simulink library "csu_tfl_thruster_forces_lander_lib"  (R2015b)
settings: Solver=ode45  StartTime=0.0  StopTime=10.0  RelTol=1e-3
values from neighbouring files (symbols this model uses):
  Bm = gim_motor_Bm    [csu_gmb_motor_prep.m]
  Jm = gim_motor_Jm    [csu_gmb_motor_prep.m]
  Ke = gim_motor_Ke    [csu_gmb_motor_prep.m]
  Kl = gim_motor_Kl    [csu_gmb_motor_prep.m]
  Kt = gim_motor_Kt    [csu_gmb_motor_prep.m]
  Lm = gim_motor_Lm    [csu_gmb_motor_prep.m]
  nb = gim_motor_nb    [csu_gmb_motor_prep.m]
  Rm = gim_motor_Rm    [csu_gmb_motor_prep.m]
undefined symbols (not defined in the file or in its folder): DiscIntNeverNeededParam, tpl_x_gimbal_actuator_to_angle, tpl_y_gimbal_actuator_to_angle
libraries: util_thruster_lib x26, util_quat_lib x2, util_info_lib x1
settings Model: Creator=Nilesh  LastModifiedBy=jimkaidy
settings DataIOCC: SaveFormat=Array
settings OptimizationCC: ExpressionDepthLimit=2147483647
settings DebuggingCC: UnderspecifiedInitializationDetection=Classic  MergeDetectMultiDrivingBlocksExec=none  SolverPrmCheckMsg=warning  StateNameClashWarn=warning
settings HardwareCC: ProdBitPerPointer=32  ProdLargestAtomicFloat=None  ProdIntDivRoundTo=Undefined  ProdEndianess=Unspecified  ProdWordSize=32  ProdHWDeviceType=32-bit Generic
settings GRTTargetCC: GeneratePreprocessorConditionals=Disable all
settings ConfigComp: CovModelRefEnable=Off  CovSFcnEnable=off

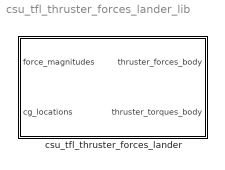
== system csu_tfl_thruster_forces_lander_lib ==
  csu_tfl_thruster_forces_lander : Subsystem

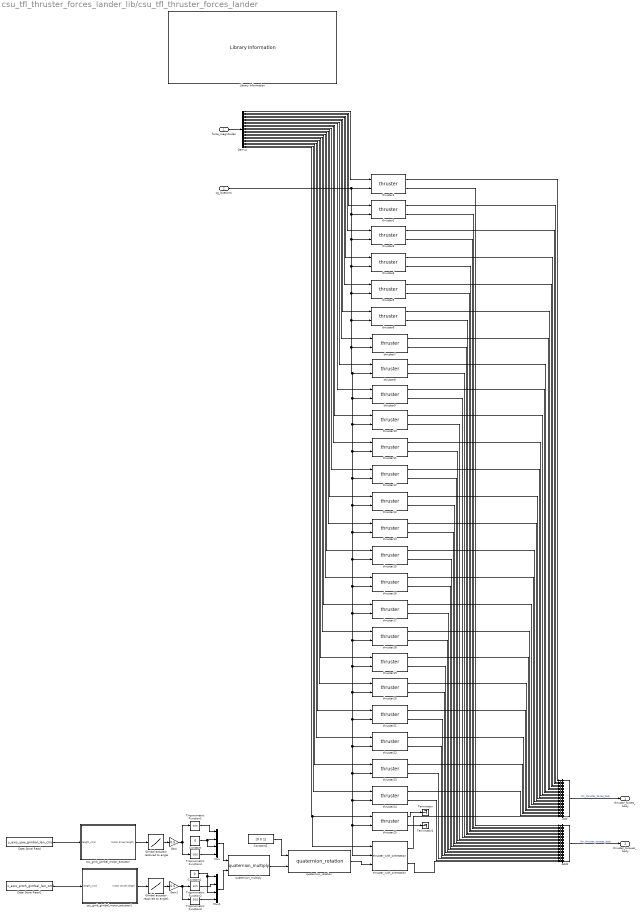
== system csu_tfl_thruster_forces_lander_lib/csu_tfl_thruster_forces_lander ==
  force_magnitudes : Inport
  cg_locations : Inport  Port=2
  Add : Sum  Inputs=+++++++++++++++++++++++++
  Add1 : Sum  Inputs=+++++++++++++++++++++++++
  Constant : Constant  Value=0
  Constant1 : Constant  Value=0
  Constant2 : Constant  Value=[0 0 1]
  Data Store Read : DataStoreRead  DataStoreName=y_axis_yaw_gimbal_len_cmd
  Data Store Read1 : DataStoreRead  DataStoreName=x_axis_pitch_gimbal_len_cmd
  Demux : Demux  Outputs=25
  Gain : Gain  Gain=0.5
  Gain1 : Gain  Gain=0.5
  Gimbal actuator resolved to angle : Lookup  InputValues=tpl_x_gimbal_actuator_to_angle(:,1)  Table=tpl_x_gimbal_actuator_to_angle(:,2)  LookUpMeth=Interpolation-Use End Values
  Gimbal actuator resolved to angle1 : Lookup  InputValues=tpl_y_gimbal_actuator_to_angle(:,1)  Table=tpl_y_gimbal_actuator_to_angle(:,2)  LookUpMeth=Interpolation-Use End Values
  Library Information : util_info_lib/Library Information  owner='NONE'
  Mux : Mux
  Mux1 : Mux
  Terminator : Terminator
  Terminator1 : Terminator
  Trigonometric Function1 : Trigonometry
  Trigonometric Function2 : Trigonometry
  Trigonometric Function3 : Trigonometry  Operator=cos
  Trigonometric Function4 : Trigonometry  Operator=cos
  csu_gmb_gimbal_motor_actuator : Subsystem
  csu_gmb_gimbal_motor_actuator1 : Subsystem
  quaternion_multiply : util_quat_lib/quaternion_multiply  SystemSampleTime=-1
  quaternion_rotation : util_quat_lib/quaternion_rotation  SystemSampleTime=-1
  thruster1 : util_thruster_lib/thruster  Thruster_Position=tfl_thruster1_position  Thruster_Orientation=tfl_thruster1_orientation
  thruster10 : util_thruster_lib/thruster  Thruster_Position=tfl_thruster10_position  Thruster_Orientation=tfl_thruster10_orientation
  thruster11 : util_thruster_lib/thruster  Thruster_Position=tfl_thruster11_position  Thruster_Orientation=tfl_thruster11_orientation
  thruster12 : util_thruster_lib/thruster  Thruster_Position=tfl_thruster12_position  Thruster_Orientation=tfl_thruster12_orientation
  thruster13 : util_thruster_lib/thruster  Thruster_Position=tfl_thruster13_position  Thruster_Orientation=tfl_thruster13_orientation
  thruster14 : util_thruster_lib/thruster  Thruster_Position=tfl_thruster14_position  Thruster_Orientation=tfl_thruster14_orientation
  thruster15 : util_thruster_lib/thruster  Thruster_Position=tfl_thruster15_position  Thruster_Orientation=tfl_thruster15_orientation
  thruster16 : util_thruster_lib/thruster  Thruster_Position=tfl_thruster16_position  Thruster_Orientation=tfl_thruster16_orientation
  thruster17 : util_thruster_lib/thruster  Thruster_Position=tfl_thruster17_position  Thruster_Orientation=tfl_thruster17_orientation
  thruster18 : util_thruster_lib/thruster  Thruster_Position=tfl_thruster18_position  Thruster_Orientation=tfl_thruster18_orientation
  thruster19 : util_thruster_lib/thruster  Thruster_Position=tfl_thruster19_position  Thruster_Orientation=tfl_thruster19_orientation
  thruster2 : util_thruster_lib/thruster  Thruster_Position=tfl_thruster2_position  Thruster_Orientation=tfl_thruster2_orientation
  thruster20 : util_thruster_lib/thruster  Thruster_Position=tfl_thruster20_position  Thruster_Orientation=tfl_thruster20_orientation
  thruster21 : util_thruster_lib/thruster  Thruster_Position=tfl_thruster21_position  Thruster_Orientation=tfl_thruster21_orientation
  thruster22 : util_thruster_lib/thruster  Thruster_Position=tfl_thruster22_position  Thruster_Orientation=tfl_thruster22_orientation
  thruster23 : util_thruster_lib/thruster  Thruster_Position=tfl_thruster23_position  Thruster_Orientation=tfl_thruster23_orientation
  thruster24 : util_thruster_lib/thruster  Thruster_Position=tfl_thruster24_position  Thruster_Orientation=tfl_thruster24_orientation
  thruster25 : util_thruster_lib/thruster  Thruster_Position=tfl_thruster25_position  Thruster_Orientation=tfl_thruster25_orientation
  thruster3 : util_thruster_lib/thruster  Thruster_Position=tfl_thruster3_position  Thruster_Orientation=tfl_thruster3_orientation
  thruster4 : util_thruster_lib/thruster  Thruster_Position=tfl_thruster4_position  Thruster_Orientation=tfl_thruster4_orientation
  thruster5 : util_thruster_lib/thruster  Thruster_Position=tfl_thruster5_position  Thruster_Orientation=tfl_thruster5_orientation
  thruster6 : util_thruster_lib/thruster  Thruster_Position=tfl_thruster6_position  Thruster_Orientation=tfl_thruster6_orientation
  thruster7 : util_thruster_lib/thruster  Thruster_Position=tfl_thruster7_position  Thruster_Orientation=tfl_thruster7_orientation
  thruster8 : util_thruster_lib/thruster  Thruster_Position=tfl_thruster8_position  Thruster_Orientation=tfl_thruster8_orientation
  thruster9 : util_thruster_lib/thruster  Thruster_Position=tfl_thruster9_position  Thruster_Orientation=tfl_thruster9_orientation
  thruster_with_orientation : util_thruster_lib/thruster_with_orientation  Thruster_Position=tfl_thruster25_position
  thruster_forces_body : Outport
  thruster_torques_body : Outport  Port=2
  wires:
  cg_locations/1 -> thruster7/2, thruster16/2, thruster18/2, thruster19/2, thruster23/2, thruster_with_orientation/2, thruster25/2, thruster24/2, thruster22/2, thruster21/2, thruster20/2, thruster17/2, thruster15/2, thruster14/2, thruster13/2, thruster12/2, thruster11/2, thruster10/2, thruster9/2, thruster8/2, thruster6/2, thruster5/2, thruster4/2, thruster3/2, thruster2/2, thruster1/2
  force_magnitudes/1 -> Demux/1
  Add1/1 -> thruster_torques_body/1  "thr_thruster_torques_body"
  thruster1/1 -> Add/1
  thruster2/1 -> Add/2
  thruster3/1 -> Add/3
  Demux/1 -> thruster1/1
  Demux/2 -> thruster2/1
  Demux/3 -> thruster3/1
  Demux/4 -> thruster4/1
  Demux/5 -> thruster5/1
  Demux/6 -> thruster6/1
  Demux/7 -> thruster7/1
  thruster1/2 -> Add1/1
  thruster2/2 -> Add1/2
  thruster3/2 -> Add1/3
  thruster4/2 -> Add1/4
  thruster5/2 -> Add1/5
  thruster6/2 -> Add1/6
  thruster7/2 -> Add1/7
  Add/1 -> thruster_forces_body/1  "thr_thruster_forces_body"
  Demux/8 -> thruster8/1
  Demux/9 -> thruster9/1
  Demux/10 -> thruster10/1
  Demux/11 -> thruster11/1
  Demux/12 -> thruster12/1
  Demux/13 -> thruster13/1
  Demux/14 -> thruster14/1
  Demux/15 -> thruster15/1
  Demux/16 -> thruster16/1
  Demux/17 -> thruster17/1
  Demux/18 -> thruster18/1
  Demux/19 -> thruster19/1
  Demux/20 -> thruster20/1
  Demux/21 -> thruster21/1
  Demux/22 -> thruster22/1
  Demux/23 -> thruster23/1
  Demux/24 -> thruster24/1
  Demux/25 -> thruster_with_orientation/1, thruster25/1
  thruster4/1 -> Add/4
  thruster5/1 -> Add/5
  thruster6/1 -> Add/6
  thruster7/1 -> Add/7
  thruster8/1 -> Add/8
  thruster9/1 -> Add/9
  thruster10/1 -> Add/10
  thruster11/1 -> Add/11
  thruster12/1 -> Add/12
  thruster13/1 -> Add/13
  thruster14/1 -> Add/14
  thruster15/1 -> Add/15
  thruster16/1 -> Add/16
  thruster17/1 -> Add/17
  thruster18/1 -> Add/18
  thruster19/1 -> Add/19
  thruster20/1 -> Add/20
  thruster21/1 -> Add/21
  thruster22/1 -> Add/22
  thruster23/1 -> Add/23
  thruster24/1 -> Add/24
  thruster_with_orientation/1 -> Add/25
  thruster8/2 -> Add1/8
  thruster9/2 -> Add1/9
  thruster10/2 -> Add1/10
  thruster11/2 -> Add1/11
  thruster12/2 -> Add1/12
  thruster13/2 -> Add1/13
  thruster14/2 -> Add1/14
  thruster15/2 -> Add1/15
  thruster16/2 -> Add1/16
  thruster17/2 -> Add1/17
  thruster18/2 -> Add1/18
  thruster19/2 -> Add1/19
  thruster20/2 -> Add1/20
  thruster21/2 -> Add1/21
  thruster22/2 -> Add1/22
  thruster23/2 -> Add1/23
  thruster24/2 -> Add1/24
  thruster_with_orientation/2 -> Add1/25
  csu_gmb_gimbal_motor_actuator/1(motor driven length) -> Gimbal actuator resolved to angle/1
  csu_gmb_gimbal_motor_actuator1/1(motor driven length) -> Gimbal actuator resolved to angle1/1
  Data Store Read1/1 -> csu_gmb_gimbal_motor_actuator1/1(length_cmd)
  Gimbal actuator resolved to angle1/1 -> Gain1/1
  Gimbal actuator resolved to angle/1 -> Gain/1
  Mux/1 -> quaternion_multiply/1
  Mux1/1 -> quaternion_multiply/2
  quaternion_multiply/1 -> quaternion_rotation/2
  Constant2/1 -> quaternion_rotation/1
  quaternion_rotation/1 -> thruster_with_orientation/3
  thruster25/2 -> Terminator1/1
  thruster25/1 -> Terminator/1
  Data Store Read/1 -> csu_gmb_gimbal_motor_actuator/1(length_cmd)
  Trigonometric Function4/1 -> Mux/4
  Constant/1 -> Mux/2, Mux/3
  Trigonometric Function2/1 -> Mux1/2
  Trigonometric Function3/1 -> Mux1/4
  Trigonometric Function1/1 -> Mux/1
  Constant1/1 -> Mux1/3, Mux1/1
  Gain/1 -> Trigonometric Function4/1, Trigonometric Function1/1
  Gain1/1 -> Trigonometric Function3/1, Trigonometric Function2/1

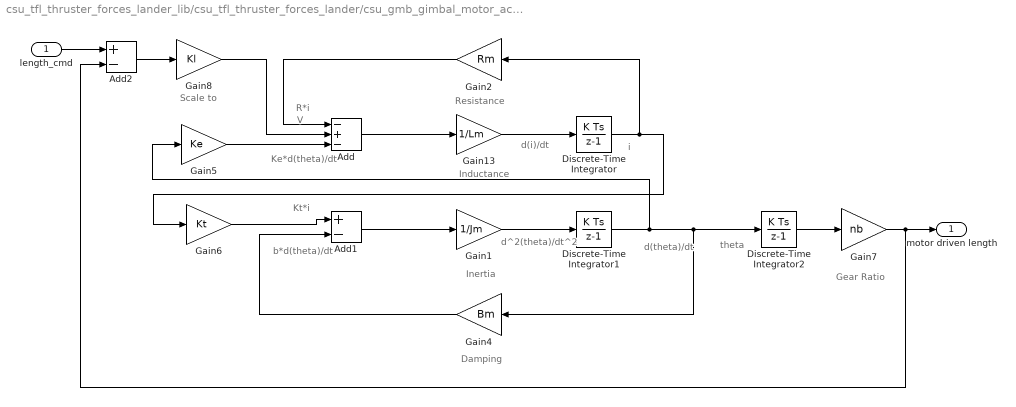
== system csu_tfl_thruster_forces_lander_lib/csu_tfl_thruster_forces_lander/csu_gmb_gimbal_motor_actuator ==
  note: Scale to
  note: theta
  note: d^2(theta)/dt^2
  note: b*d(theta)/dt
  note: Kt*i
  note: d(theta)/dt
  note: Ke*d(theta)/dt
  note: V
  note: R*i
  note: i
  note: d(i)/dt
  note: Gear Ratio
  note: Resistance
  note: Damping
  note: Inertia
  note: Inductance
  length_cmd : Inport
  Add : Sum  Inputs=-+-
  Add1 : Sum  Inputs=+-
  Add2 : Sum  Inputs=+-
  Discrete-Time Integrator : DiscreteIntegrator  InitialConditionSetting=State (most efficient)  SampleTime=-1  ICPrevOutput=DiscIntNeverNeededParam  ICPrevScaledInput=DiscIntNeverNeededParam
  Discrete-Time Integrator1 : DiscreteIntegrator  InitialConditionSetting=State (most efficient)  SampleTime=-1  ICPrevOutput=DiscIntNeverNeededParam  ICPrevScaledInput=DiscIntNeverNeededParam
  Discrete-Time Integrator2 : DiscreteIntegrator  InitialConditionSetting=State (most efficient)  SampleTime=-1  ICPrevOutput=DiscIntNeverNeededParam  ICPrevScaledInput=DiscIntNeverNeededParam
  Gain1 : Gain  Gain=1/Jm
  Gain13 : Gain  Gain=1/Lm
  Gain2 : Gain  Gain=Rm
  Gain4 : Gain  Gain=Bm
  Gain5 : Gain  Gain=Ke
  Gain6 : Gain  Gain=Kt
  Gain7 : Gain  Gain=nb
  Gain8 : Gain  Gain=Kl
  motor driven length : Outport
  wires:
  length_cmd/1 -> Add2/1
  Gain13/1 -> Discrete-Time Integrator/1
  Gain1/1 -> Discrete-Time Integrator1/1
  Gain5/1 -> Add/3
  Gain4/1 -> Add1/2
  Gain2/1 -> Add/1
  Gain6/1 -> Add1/1
  Discrete-Time Integrator/1 -> Gain2/1, Gain6/1
  Gain8/1 -> Add/2
  Add/1 -> Gain13/1
  Add1/1 -> Gain1/1
  Discrete-Time Integrator1/1 -> Gain5/1, Gain4/1, Discrete-Time Integrator2/1
  Add2/1 -> Gain8/1
  Discrete-Time Integrator2/1 -> Gain7/1
  Gain7/1 -> Add2/2, motor driven length/1

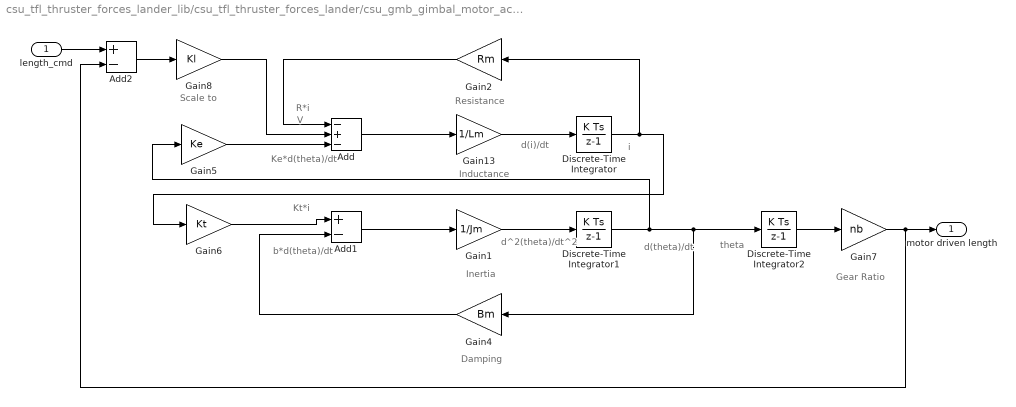
== system csu_tfl_thruster_forces_lander_lib/csu_tfl_thruster_forces_lander/csu_gmb_gimbal_motor_actuator1 ==
  note: Scale to
  note: theta
  note: d^2(theta)/dt^2
  note: b*d(theta)/dt
  note: Kt*i
  note: d(theta)/dt
  note: Ke*d(theta)/dt
  note: V
  note: R*i
  note: i
  note: d(i)/dt
  note: Gear Ratio
  note: Resistance
  note: Damping
  note: Inertia
  note: Inductance
  length_cmd : Inport
  Add : Sum  Inputs=-+-
  Add1 : Sum  Inputs=+-
  Add2 : Sum  Inputs=+-
  Discrete-Time Integrator : DiscreteIntegrator  InitialConditionSetting=State (most efficient)  SampleTime=-1  ICPrevOutput=DiscIntNeverNeededParam  ICPrevScaledInput=DiscIntNeverNeededParam
  Discrete-Time Integrator1 : DiscreteIntegrator  InitialConditionSetting=State (most efficient)  SampleTime=-1  ICPrevOutput=DiscIntNeverNeededParam  ICPrevScaledInput=DiscIntNeverNeededParam
  Discrete-Time Integrator2 : DiscreteIntegrator  InitialConditionSetting=State (most efficient)  SampleTime=-1  ICPrevOutput=DiscIntNeverNeededParam  ICPrevScaledInput=DiscIntNeverNeededParam
  Gain1 : Gain  Gain=1/Jm
  Gain13 : Gain  Gain=1/Lm
  Gain2 : Gain  Gain=Rm
  Gain4 : Gain  Gain=Bm
  Gain5 : Gain  Gain=Ke
  Gain6 : Gain  Gain=Kt
  Gain7 : Gain  Gain=nb
  Gain8 : Gain  Gain=Kl
  motor driven length : Outport
  wires:
  length_cmd/1 -> Add2/1
  Gain13/1 -> Discrete-Time Integrator/1
  Gain1/1 -> Discrete-Time Integrator1/1
  Gain5/1 -> Add/3
  Gain4/1 -> Add1/2
  Gain2/1 -> Add/1
  Gain6/1 -> Add1/1
  Discrete-Time Integrator/1 -> Gain2/1, Gain6/1
  Gain8/1 -> Add/2
  Add/1 -> Gain13/1
  Add1/1 -> Gain1/1
  Discrete-Time Integrator1/1 -> Gain5/1, Gain4/1, Discrete-Time Integrator2/1
  Add2/1 -> Gain8/1
  Discrete-Time Integrator2/1 -> Gain7/1
  Gain7/1 -> Add2/2, motor driven length/1
